simulink library "CalcMinDist"  (R2018b)
settings: Solver=VariableStepAuto  StartTime=0.0  StopTime=10.0  RelTol=1e-3
libraries: simulink x2
settings Model: Creator=BI28030  LastModifiedBy=BI28030

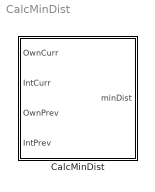
== system CalcMinDist ==
  CalcMinDist : Subsystem  mask(CalcMinDist){}
      mask help:
      | Calculate the minimum distance between two points moving at constant
      | velocity between the given previous and current locations
      | in R^n Euclidean space

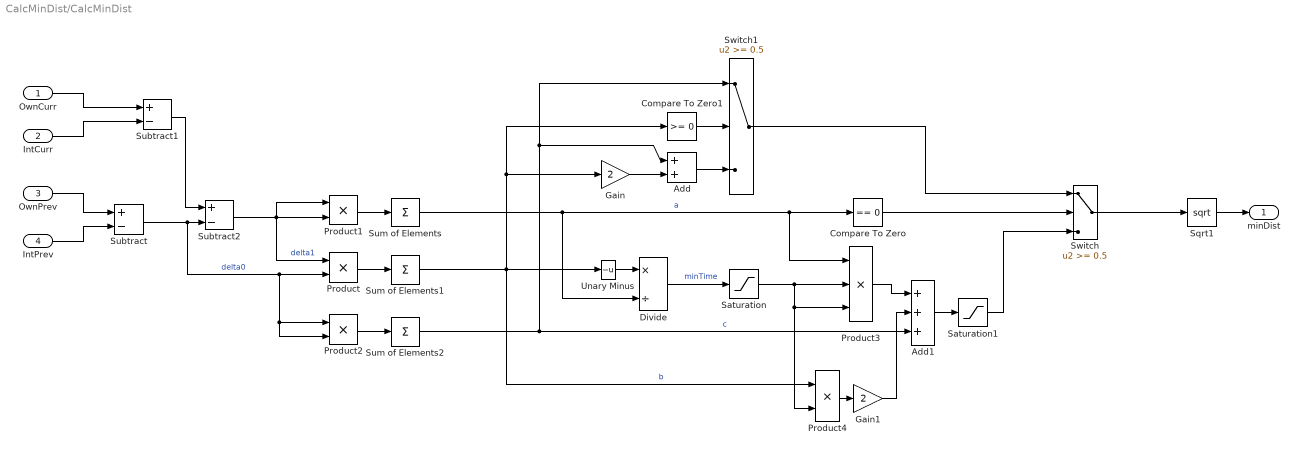
== system CalcMinDist/CalcMinDist ==
  OwnCurr : Inport
  IntCurr : Inport  Port=2
  OwnPrev : Inport  Port=3
  IntPrev : Inport  Port=4
  Add : Sum
  Add1 : Sum  Inputs=+++
  Compare To Zero : simulink/Logic and Bit Operations/Compare To Zero  relop===  OutDataTypeStr=boolean
  Compare To Zero1 : simulink/Logic and Bit Operations/Compare To Zero  relop=>=  OutDataTypeStr=boolean
  Divide : Product  Inputs=*/
  Gain : Gain  Gain=2
  Gain1 : Gain  Gain=2
  Product{,1..2,4} (4 alike) : Product
  Product3 : Product  Inputs=3
  Saturation : Saturate  UpperLimit=1  LowerLimit=0
  Saturation1 : Saturate  UpperLimit=inf  LowerLimit=0
  Sqrt1 : Sqrt  SaturateOnIntegerOverflow=on
  Subtract : Sum  Inputs=+-
  Subtract1 : Sum  Inputs=+-
  Subtract2 : Sum  Inputs=+-
  Sum of Elements : Sum  Inputs=+
  Sum of Elements1 : Sum  Inputs=+
  Sum of Elements2 : Sum  Inputs=+
  Switch : Switch  Threshold=0.5
  Switch1 : Switch  Threshold=0.5
  Unary Minus : UnaryMinus
  minDist : Outport
  wires:
  Saturation1/1 -> Switch/3
  OwnPrev/1 -> Subtract/1
  IntPrev/1 -> Subtract/2
  IntCurr/1 -> Subtract1/2
  OwnCurr/1 -> Subtract1/1
  Subtract1/1 -> Subtract2/1
  Subtract/1 -> Product2/2, Product2/1, Product/2, Subtract2/2  "delta0"
  Subtract2/1 -> Product1/1, Product1/2, Product/1  "delta1"
  Product1/1 -> Sum of Elements/1
  Product/1 -> Sum of Elements1/1
  Product2/1 -> Sum of Elements2/1
  Sum of Elements/1 -> Divide/2, Product3/1, Compare To Zero/1  "a"
  Sum of Elements1/1 -> Product4/1, Unary Minus/1, Gain/1, Compare To Zero1/1  "b"
  Sum of Elements2/1 -> Switch1/1, Add/1, Add1/3  "c"
  Compare To Zero/1 -> Switch/2
  Compare To Zero1/1 -> Switch1/2
  Switch1/1 -> Switch/1
  Add/1 -> Switch1/3
  Gain/1 -> Add/2
  Unary Minus/1 -> Divide/1
  Divide/1 -> Saturation/1  "minTime"
  Saturation/1 -> Product3/3, Product4/2, Product3/2
  Product3/1 -> Add1/1
  Add1/1 -> Saturation1/1
  Product4/1 -> Gain1/1
  Switch/1 -> Sqrt1/1
  Sqrt1/1 -> minDist/1
  Gain1/1 -> Add1/2
